simulink model "furuta_pend_mimic_live"  (R2013a)
settings: Solver=ode3  StartTime=0.0  StopTime=20  FixedStep=.001  RelTol=1e-3
undefined symbols (not defined in the file or in its folder): energy_SMC_controller_sim, furuta_state_derivatives
settings Model: Creator=Holly Warner  LastModifiedBy=Holly Warner

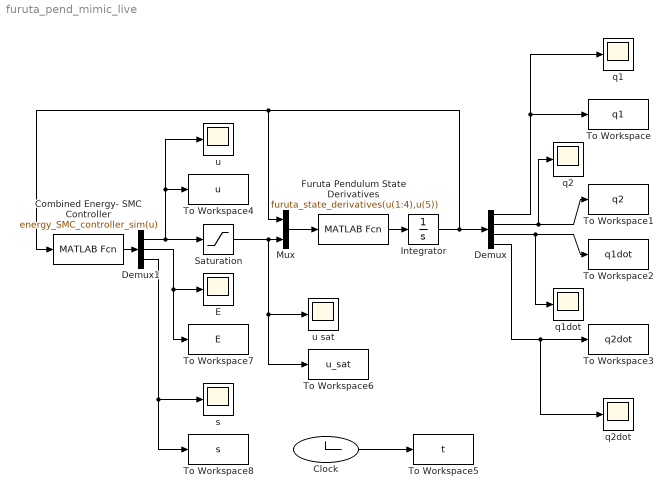
== system furuta_pend_mimic_live ==
  Clock : Clock
  Combined Energy- SMC Controller : MATLABFcn  MATLABFcn=energy_SMC_controller_sim(u)  OutputDimensions=3
  Demux : Demux
  Demux1 : Demux  Outputs=3
  E : Scope
      settings: TimeRange=2  YMin=-0.25  YMax=1.38778e-17  SaveName=ScopeData3
  Furuta Pendulum State Derivatives : MATLABFcn  MATLABFcn=furuta_state_derivatives(u(1:4),u(5))
  Integrator : Integrator  InitialCondition=[0 pi 0 0]
  Mux : Mux  Inputs=2
  Saturation : Saturate  UpperLimit=4.5  LowerLimit=-4.5
  To Workspace : ToWorkspace  VariableName=q1  SampleTime=-1
  To Workspace1 : ToWorkspace  VariableName=q2  SampleTime=-1
  To Workspace2 : ToWorkspace  VariableName=q1dot  SampleTime=-1
  To Workspace3 : ToWorkspace  VariableName=q2dot  SampleTime=-1
  To Workspace4 : ToWorkspace  VariableName=u  SampleTime=-1
  To Workspace5 : ToWorkspace  VariableName=t  SampleTime=-1
  To Workspace6 : ToWorkspace  VariableName=u_sat  SampleTime=-1
  To Workspace7 : ToWorkspace  VariableName=E  SampleTime=-1
  To Workspace8 : ToWorkspace  VariableName=s  SampleTime=-1
  q1 : Scope
      settings: YMin=0  YMax=1.1
  q1dot : Scope
      settings: YMin=-6  YMax=2  SaveName=ScopeData5
  q2 : Scope
      settings: TimeRange=5  YMin=-1.32025e-09  YMax=-1.31675e-09  SaveName=ScopeData2
  q2dot : Scope
      settings: YMin=-1  YMax=0.5  SaveName=ScopeData6
  s : Scope
      settings: YMin=-32.5  YMax=2.5  SaveName=ScopeData4
  u : Scope
      settings: TimeRange=20  YMin=-100  YMax=175
  u sat : Scope
      settings: TimeRange=20  SaveName=ScopeData7
  wires:
  Demux/1 -> To Workspace/1, q1/1
  Demux/2 -> To Workspace1/1, q2/1
  Demux/3 -> To Workspace2/1, q1dot/1
  Demux/4 -> q2dot/1, To Workspace3/1
  Furuta Pendulum State Derivatives/1 -> Integrator/1
  Mux/1 -> Furuta Pendulum State Derivatives/1
  Integrator/1 -> Combined Energy- SMC Controller/1, Mux/1, Demux/1
  Combined Energy- SMC Controller/1 -> Demux1/1
  Demux1/1 -> u/1, To Workspace4/1, Saturation/1
  Demux1/2 -> E/1, To Workspace7/1
  Demux1/3 -> To Workspace8/1, s/1
  Clock/1 -> To Workspace5/1
  Saturation/1 -> u sat/1, To Workspace6/1, Mux/2
